simulink model "fir_fixed_test"  (R2014b)
settings: Solver=ode45  StartTime=0.0  StopTime=inf  RelTol=1e-3
libraries: simulink x1
settings Model: Creator=Ben  LastModifiedBy=Ben

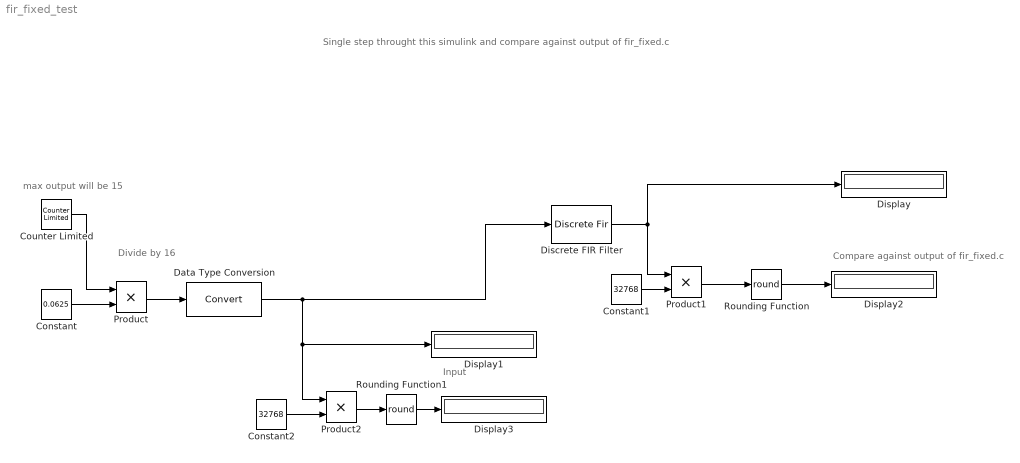
== system fir_fixed_test ==
  note: Single step throught this simulink and compare against output of fir_fixed.c
  note: Input
  note: Compare against output of fir_fixed.c
  note: max output will be 15
  note: Divide by 16
  Constant : Constant  Value=0.0625
  Constant1 : Constant  Value=32768
  Constant2 : Constant  Value=32768
  Counter Limited : simulink/Sources/Counter Limited  uplimit=15  tsamp=1/125E3
  Data Type Conversion : DataTypeConversion  RndMeth=Nearest
  Discrete FIR Filter : DiscreteFir  Coefficients=[.04 .05 .03]
  Display{,1..3} (4 alike) : Display
  Product : Product
  Product1 : Product
  Product2 : Product
  Rounding Function : Rounding  Operator=round
  Rounding Function1 : Rounding  Operator=round
  wires:
  Discrete FIR Filter/1 -> Product1/1, Display/1
  Data Type Conversion/1 -> Discrete FIR Filter/1, Product2/1, Display1/1
  Counter Limited/1 -> Product/1
  Product/1 -> Data Type Conversion/1
  Constant/1 -> Product/2
  Product1/1 -> Rounding Function/1
  Rounding Function/1 -> Display2/1
  Constant1/1 -> Product1/2
  Product2/1 -> Rounding Function1/1
  Constant2/1 -> Product2/2
  Rounding Function1/1 -> Display3/1
